simulink model "DemoPlant"  (R2024b)
settings: Solver=VariableStepAuto  StartTime=0.0  StopTime=10.0  RelTol=1e-3
settings Model: DataDictionary=Data.sldd  Creator=toma  LastModifiedBy=toma
settings ModelReferenceCC: UpdateModelReferenceTargets=IfOutOfDate
settings ConfigComp: CovBoundaryAbsTol=1.0e-5

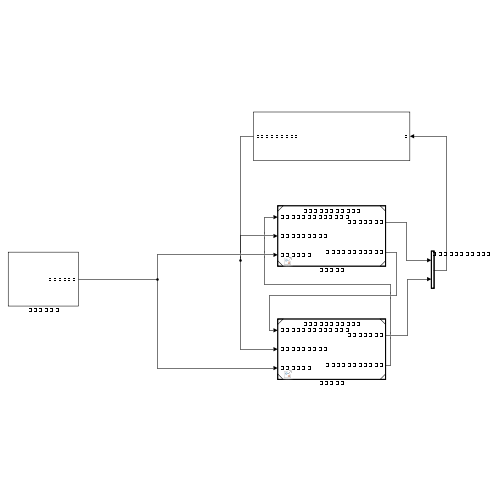
[thumbnail: Simulink's stored preview of the top-level diagram]
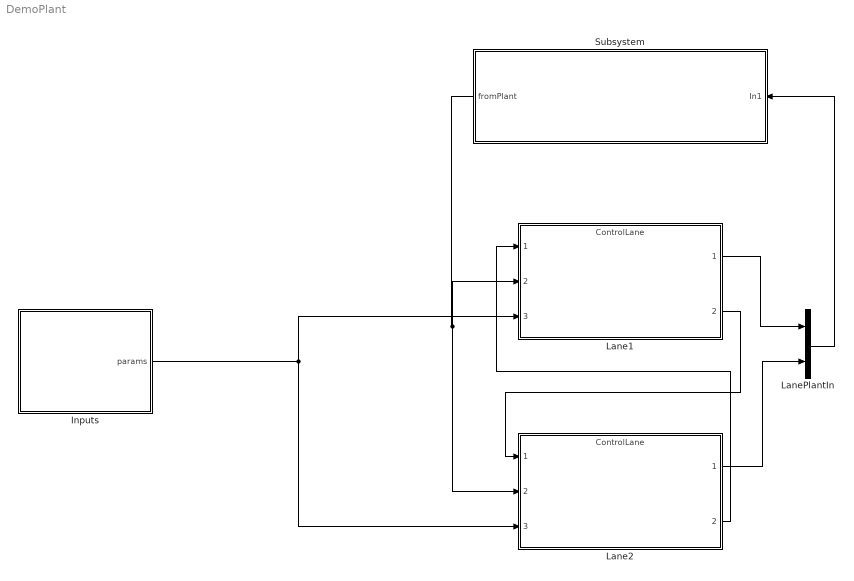
== system DemoPlant ==
  Inputs : Subsystem
  Lane1 : ModelReference  ModelNameDialog=ControlLane  SimulationMode=Normal  ModelReferenceVersion=1.7
  Lane2 : ModelReference  ModelNameDialog=ControlLane  SimulationMode=Normal  ModelReferenceVersion=1.7
  LanePlantIn : BusCreator  Inputs=2  OutDataTypeStr=Bus: PlantInBundle
  Subsystem : Subsystem
  wires:
  Inputs/1(params) -> Lane2/3, Lane1/3
  Subsystem/1(fromPlant) -> Lane2/2, Lane1/2
  Lane1/1 -> LanePlantIn/1
  Lane2/1 -> LanePlantIn/2
  LanePlantIn/1 -> Subsystem/1(In1)
  Lane1/2 -> Lane2/1
  Lane2/2 -> Lane1/1

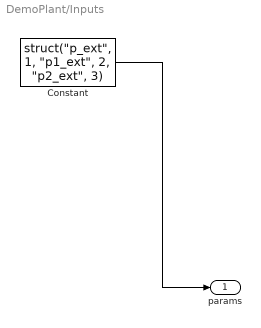
== system DemoPlant/Inputs ==
  Constant : Constant  Value="struct(\"p_ext\", 1, \"p1_ext\", 2, \"p2_ext\", 3)"  OutDataTypeStr=Bus: ExtParams
  params : Outport
  wires:
  Constant/1 -> params/1

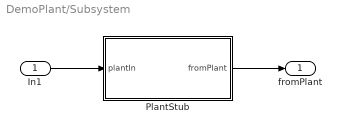
== system DemoPlant/Subsystem ==
  In1 : Inport  OutDataTypeStr=Bus: PlantInBundle
  PlantStub : MATLAB Function  TreatAsAtomicUnit=on
  fromPlant : Outport  OutDataTypeStr=Bus: PlantOut
  wires:
  In1/1 -> PlantStub/1(plantIn)
  PlantStub/1(fromPlant) -> fromPlant/1

== matlab function DemoPlant/Subsystem/PlantStub ==
  data: plantIn input Bus: PlantInBundle; fromPlant output Bus: PlantOut
function fromPlant = fcn(plantIn)

fromPlant.a_p = plantIn.lane1.pOut.a_p;
fromPlant.a1_p = plantIn.lane1.pOut.a1_p;
fromPlant.a2_p = plantIn.lane1.pOut.a2_p;

end
